simulink model "QPSKMODEM"  (R2020b)
settings: Solver=VariableStepAuto  StartTime=0.0  StopTime=inf  RelTol=1e-3
model workspace (MAT data in the model file):
  BitRate = 20480
  CoreFreq = 40960
  RCF_Rolloff_factor = 0.1
  SampleRateQPSK = 819200
undefined symbols (not defined in the file): fdesignblkfcn, gcbh, random
libraries: simulink_extras x9, simulink x6, commfilt2 x4, dspsrcs4 x3, commrfcorlib x2, commutil2 x2, dspmathops x2, commrandsrc3 x1, commsink2 x1, commchan3 x1
(part 1 of 2)
settings Model: OrderedModelArguments=off  Creator=Unknown Username  LastModifiedBy=AlexKurash
settings DataIOCC: ReturnWorkspaceOutputs=off
settings DebuggingCC: ParameterOverflowMsg=none  ArithmeticOperatorsInVariantConditions=warning
settings SFSimCC: SimUseLocalCustomCode=off  CustomCodeUndefinedFunction=UseInterfaceOnly
settings RTWCC: RTWUseLocalCustomCode=off

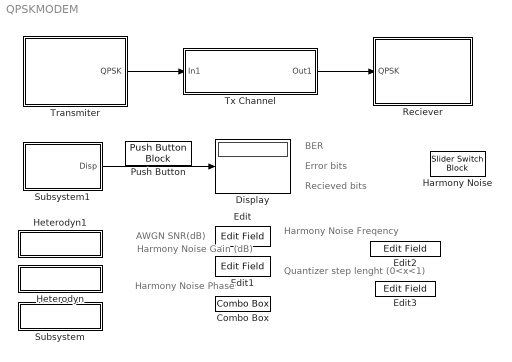
== system QPSKMODEM ==
  note: BER
  note: Error bits
  note: Recieved bits
  note: AWGN SNR(dB)
  note: Harmony Noise
      | Gain (dB)
  note: Harmony Noise
      | Phase
  note: Harmony Noise
      | Freqency
  note: Quantizer step lenght (0<x<1)
  Combo Box : ComboBox  LabelPosition=Hide  SelectedLabel=45deg
      settings: Values={{'0deg', '10deg', '20deg', '30deg', '45deg', '90deg', '180deg'}, [0 0.174533 0.349066 0.523598 0.785398 1.570796 3.141592]}
  Display : Display
  Edit{,1..3} (4 alike) : EditField  LabelPosition=Hide  ShowInitialText=on  Alignment=Center
  Harmony Noise : SliderSwitchBlock
      settings: Values={{'Off', 'On'}, [0 1]}
  Heterodyn : Subsystem
      mask Display:
      | color('red');
      | disp('Heterodyn')
  Heterodyn1 : Subsystem
      mask Display:
      | color('red');
      | disp('Syncronization')
  Push Button : PushButtonBlock  ButtonText=RESET
  Reciever : Subsystem
      mask Display:
      | color('purple');
      | disp('OQPSK \n RECIEVER')
      | color('black');
  Subsystem : Subsystem
      mask Display:
      | color('red');
      | disp('Dbit Generator')
  Subsystem1 : Subsystem
      mask Display:
      | color('red')
      | 
      | disp('Graphics\n and \n BER calculation')
  Transmiter : Subsystem
      mask Display:
      | color('blue');
      | disp('OQPSK \n TRANSMITER')
      | color('black');
  Tx Channel : Subsystem
      mask Display:
      | plot(-10,-10,110, 110,[05 15 10 10 05 10 18 14 13 7.5 13 41 44 47 50 53 57 ...
      | 59 100-[13 7.5 13 14 18 10 5 10 10 15 5]],[70 70 70 85 92 85 79 82 90 88.5 ...
      | 90 90 87 93 87 93 87 90 90 88.5 90 82 79 85 92 85 70 70 70]);
      | disp('CHANNEL');
  wires:
  Subsystem1/1(Disp) -> Display/1
  Transmiter/1(QPSK) -> Tx Channel/1(In1)
  Tx Channel/1(Out1) -> Reciever/1(QPSK)

== system QPSKMODEM/Heterodyn ==
  Local Oscillator : dspsrcs4/Sine Wave  Amplitude=0.707  Frequency=CoreFreq  Phase=pi/2  SampleMode=Discrete  OutComplex=Real  CompMethod=Trigonometric fcn  TableSize=Speed  SampleTime=1/SampleRateQPSK  SamplesPerFrame=1  ResetState=Restart at time zero  OutputFrames=off  dataType=double  wordLen=16  udDataType=sfix(16)  fracBitsMode=Best precision  numFracBits=15  OutDataTypeStr=double  LastOutDataTypeStr=double
  Local Oscillator1 : dspsrcs4/Sine Wave  Amplitude=0.707  Frequency=CoreFreq  Phase=0  SampleMode=Discrete  OutComplex=Real  CompMethod=Trigonometric fcn  TableSize=Speed  SampleTime=1/SampleRateQPSK  SamplesPerFrame=1  ResetState=Restart at time zero  OutputFrames=off  dataType=double  wordLen=16  udDataType=sfix(16)  fracBitsMode=Best precision  numFracBits=15  OutDataTypeStr=double  LastOutDataTypeStr=double
  tag scope: Heterodyn_COS=global, Heterodyn_SIN=global
  wires:
  Local Oscillator/1 -> [Heterodyn_COS]
  Local Oscillator1/1 -> [Heterodyn_SIN]

== system QPSKMODEM/Heterodyn1 ==
  Clock : simulink_extras/Flip Flops/Clock  period=2/BitRate
  tag scope: CLK=global
  wires:
  Clock/1 -> [CLK]

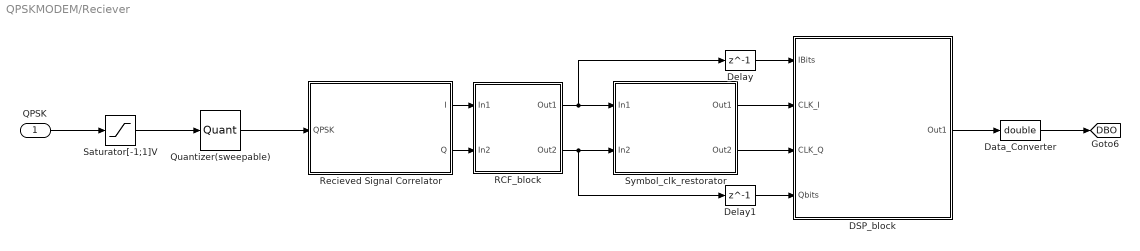
== system QPSKMODEM/Reciever ==
  QPSK : Inport
  DSP_block : Subsystem
      mask Display:
      | color('red');
      | disp('Digital \n Signal \n Processing')
      | color('black');
      | port_label('input',3,'CLK_Q')
      | port_label('input',2,'CLK_I')
      | port_label('input',1,'I_bits')
      | port_label('input',4,'Q_bits')
      | port_label('output',1,'DBit_code')
  Data_Converter : DataTypeConversion  OutDataTypeStr=double
  Delay : Delay  DelayLength=1  InitialCondition=0  SampleTime=1/BitRate
  Delay1 : Delay  DelayLength=1  InitialCondition=0  SampleTime=1/BitRate
  Quantizer(sweepable) : Quantizer  QuantizationInterval=1/8  LinearizeAsGain=off
  RCF_block : Subsystem
      mask Display:
      | color('red');
      | disp('Filtration')
      | color('black');
      | port_label('input',1,'I')
      | port_label('input',2,'Q')
      | port_label('output',1,'I')
      | port_label('output',2,'Q')
  "Recieved Signal Correlator " : Subsystem
      mask Display:
      | color('red');
      | disp('Correlation')
      | color('black');
      | port_label('input',1,'OPSK')
      | port_label('output',1,'I')
      | port_label('output',2,'Q')
  Saturator[-1;1]V : Saturate  UpperLimit=1  LowerLimit=-1
  Symbol_clk_restorator : Subsystem
      mask Display:
      | color('red');
      | disp('Syncronization \n restoration')
      | color('black');
      | port_label('input',1,'s(t_I)')
      | port_label('output',1,'CLK_I')
      | 
      | port_label('input',2,'s(t_Q)')
      | port_label('output',2,'CLK_Q')
  tag scope: DBO=global
  wires:
  Data_Converter/1 -> [DBO]
  "Recieved Signal Correlator "/1(I) -> RCF_block/1(In1)
  "Recieved Signal Correlator "/2(Q) -> RCF_block/2(In2)
  RCF_block/1(Out1) -> Delay/1, Symbol_clk_restorator/1(In1)
  RCF_block/2(Out2) -> Delay1/1, Symbol_clk_restorator/2(In2)
  Symbol_clk_restorator/1(Out1) -> DSP_block/2(CLK_I)
  Symbol_clk_restorator/2(Out2) -> DSP_block/3(CLK_Q)
  Delay/1 -> DSP_block/1(IBits)
  Delay1/1 -> DSP_block/4(Qbits)
  Saturator[-1;1]V/1 -> Quantizer(sweepable)/1
  DSP_block/1(Out1) -> Data_Converter/1
  Quantizer(sweepable)/1 -> "Recieved Signal Correlator "/1(QPSK)
  QPSK/1 -> Saturator[-1;1]V/1

== system QPSKMODEM/Subsystem ==
  Bernoulli Binary Generator : commrandsrc3/Bernoulli Binary Generator  ProbabilityOfZero=0.5  SeedSource=Auto  Seed=random  SampleTime=1/BitRate  SamplesPerFrame=1  OutputDataType=double  SimulateUsing=Interpreted execution
  tag scope: DB=global
  wires:
  Bernoulli Binary Generator/1 -> [DB]

== system QPSKMODEM/Subsystem1 ==
  Reciever : Subsystem
      mask Display: disp('Transmitter \n Diagrams')
  Subsystem : Subsystem
      mask Display: disp('BER \n Calculation')
  Transmiter : Subsystem
      mask Display: disp('Reciever \n Diagrams')
  spectre : Subsystem
      mask Display: disp('Signals\nSpectrum')
  spectre1 : Subsystem
      mask Display: disp('Constellation \n Diagramm')
  Disp : Outport  VectorParamsAs1DForOutWhenUnconnected=off
  wires:
  Subsystem/1(Out1) -> Disp/1

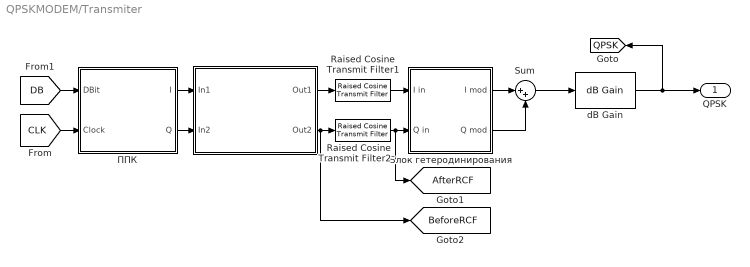
== system QPSKMODEM/Transmiter ==
  " " : Subsystem
      mask Display:
      | color('red');
      | disp('Signal Level \n Coder')
      | color('black');
      | port_label('input',1,'Odd_in')
      | port_label('input',2,'Even_in')
      | port_label('output',1,'Odd_out')
      | port_label('output',2,'Even_out')
  Raised Cosine Transmit Filter1 : commfilt2/Raised Cosine Transmit Filter  filtType=Square root  R=RCF_Rolloff_factor  filtSpan=10  N=(SampleRateQPSK/BitRate)/4  filterGain=3  RateOptions=Allow multirate processing  framing=Mute  checkCoeff=off  variableName=rcTxFilt1  checkGain=Normalized  sampMode=Mute  saveAsFlag=0  currentFiltSpan=10  D=(10)/2  launchFVT=on  roundingMode=Floor  overflowMode=off  coeffDataTypeStr=Inherit: Same word length as input  coeffMin=[]  coeffMax=[]  coeffLastDataTypeStr=Inherit: Same word length as input  outputDataTypeStr=Inherit: Same as accumulator  outputMin=[]  outputMax=[]  outputLastDataTypeStr=Inherit: Same as accumulator
  Raised Cosine Transmit Filter2 : commfilt2/Raised Cosine Transmit Filter  filtType=Square root  R=RCF_Rolloff_factor  filtSpan=10  N=(SampleRateQPSK/BitRate)/4  filterGain=3  RateOptions=Allow multirate processing  framing=Mute  checkCoeff=off  variableName=rcTxFilt2  checkGain=Normalized  sampMode=Mute  saveAsFlag=0  currentFiltSpan=10  D=(10)/2  launchFVT=on  roundingMode=Floor  overflowMode=off  coeffDataTypeStr=Inherit: Same word length as input  coeffMin=[]  coeffMax=[]  coeffLastDataTypeStr=Inherit: Same word length as input  outputDataTypeStr=Inherit: Same as accumulator  outputMin=[]  outputMax=[]  outputLastDataTypeStr=Inherit: Same as accumulator
  Sum : Sum  Inputs=|++
  dB Gain : dspmathops/dB Gain  dB=5  intype=Power
      settings: SourceProductBaseCode=DS
  "Блок гетеродинирования " : Subsystem
      mask Display:
      | color('red');
      | disp('Hyterodination')
      | color('black');
      | port_label('input',1,'Odd')
      | port_label('input',2,'Even')
      | port_label('output',1,'I')
      | port_label('output',2,'Q')
  ППК : Subsystem
      mask Display:
      | color('red');
      | disp('Serial-to-Parallel')
      | color('black');
      | port_label('input',1,'Dbit')
      | port_label('input',2,'CLK')
      | port_label('output',1,'Odd')
      | port_label('output',2,'Even')
  QPSK : Outport  VectorParamsAs1DForOutWhenUnconnected=off
  tag scope: AfterRCF=global, BeforeRCF=global, QPSK=global
  wires:
  [DB] -> ППК/1(DBit)
  [CLK] -> ППК/2(Clock)
  ППК/1(I) -> " "/1(In1)
  ППК/2(Q) -> " "/2(In2)
  "Блок гетеродинирования "/1(I mod) -> Sum/1
  "Блок гетеродинирования "/2(Q mod) -> Sum/2
  " "/1(Out1) -> Raised Cosine Transmit Filter1/1
  " "/2(Out2) -> [BeforeRCF], Raised Cosine Transmit Filter2/1
  Raised Cosine Transmit Filter1/1 -> "Блок гетеродинирования "/1(I in)
  Raised Cosine Transmit Filter2/1 -> [AfterRCF], "Блок гетеродинирования "/2(Q in)
  dB Gain/1 -> QPSK/1, [QPSK]
  Sum/1 -> dB Gain/1

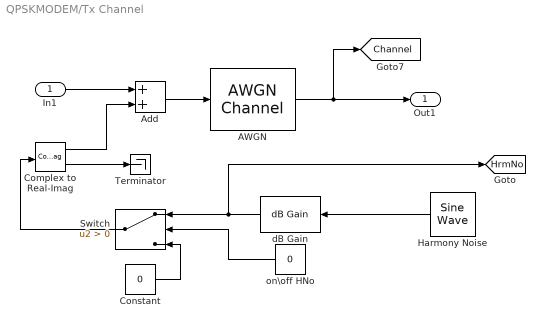
== system QPSKMODEM/Tx Channel ==
  In1 : Inport
  AWGN : commchan3/AWGN Channel  InputProcessing=Columns as channels (frame based)  seed=1  noiseMode="Signal to noise ratio  (SNR)"  EbNodB=20  EsNodB=10  SNRdB=20  bitsPerSym=2  Ps=200  Tsym=0.5/BitRate  variance=1
  Add : Sum
  Complex to Real-Imag : ComplexToRealImag
  Constant : Constant  Value=0
  Harmony Noise : dspsrcs4/Sine Wave  Amplitude=0.707  Frequency=41000  Phase=0.785398  SampleMode=Discrete  OutComplex=Real  CompMethod=Trigonometric fcn  TableSize=Speed  SampleTime=1/SampleRateQPSK  SamplesPerFrame=1  ResetState=Restart at time zero  OutputFrames=off  dataType=double  wordLen=16  udDataType=sfix(16)  fracBitsMode=Best precision  numFracBits=15  OutDataTypeStr=double  LastOutDataTypeStr=double
  Switch : Switch  Criteria=u2 > Threshold
  Terminator : Terminator
  dB Gain : dspmathops/dB Gain  dB=0  intype=Power
      settings: SourceProductBaseCode=DS
  on\off HNo : Constant  Value=0
  Out1 : Outport
  tag scope: Channel=global, HrmNo=global
  wires:
  dB Gain/1 -> [HrmNo], Switch/1
  on\off HNo/1 -> Switch/2
  In1/1 -> Add/1
  Add/1 -> AWGN/1
  Switch/1 -> Complex to Real-Imag/1
  AWGN/1 -> [Channel], Out1/1
  Complex to Real-Imag/1 -> Add/2
  Harmony Noise/1 -> dB Gain/1
  Complex to Real-Imag/2 -> Terminator/1
  Constant/1 -> Switch/3

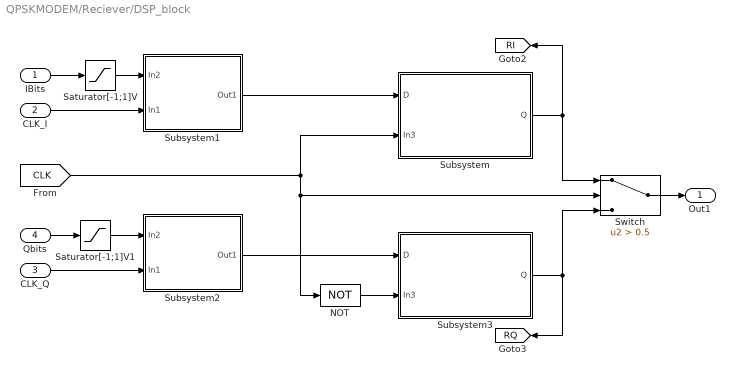
== system QPSKMODEM/Reciever/DSP_block ==
  IBits : Inport
  CLK_I : Inport  Port=2
  CLK_Q : Inport  Port=3
  Qbits : Inport  Port=4
  NOT : Logic  Operator=NOT  AllPortsSameDT=off  OutDataTypeStr=boolean
  Saturator[-1;1]V : Saturate  UpperLimit=1  LowerLimit=-1
  Saturator[-1;1]V1 : Saturate  UpperLimit=1  LowerLimit=-1
  Subsystem : Subsystem
      mask Display:
      | color('red');
      | disp('Bits \n Restoration \n device')
      | color('black');
      | port_label('output',1,'Bits')
      | port_label('input',1,'s(t)')
      | port_label('input',2,'CLK')
  Subsystem1 : Subsystem
      mask Display:
      | color('red');
      | disp('Treshold \n decision \n device')
      | color('black');
      | port_label('output',1,'Bits')
      | port_label('input',1,'s(t)')
      | port_label('input',2,'CLK')
  Subsystem2 : Subsystem
      mask Display:
      | color('red');
      | disp('Treshold \n decision \n device')
      | color('black');
      | port_label('output',1,'Bits')
      | port_label('input',1,'s(t)')
      | port_label('input',2,'CLK')
  Subsystem3 : Subsystem
      mask Display:
      | color('red');
      | disp('Bits \n Restoration \n device')
      | color('black');
      | port_label('output',1,'Bits')
      | port_label('input',1,'s(t)')
      | port_label('input',2,'CLK')
  Switch : Switch  Criteria=u2 > Threshold  Threshold=0.5
  Out1 : Outport
  tag scope: RI=global, RQ=global
  wires:
  Subsystem1/1(Out1) -> Subsystem/1(D)
  Subsystem2/1(Out1) -> Subsystem3/1(D)
  CLK_I/1 -> Subsystem1/2(In1)
  Subsystem3/1(Q) -> Switch/3, [RQ]
  Switch/1 -> Out1/1
  IBits/1 -> Saturator[-1;1]V/1
  Qbits/1 -> Saturator[-1;1]V1/1
  NOT/1 -> Subsystem3/2(In3)
  CLK_Q/1 -> Subsystem2/2(In1)
  [CLK] -> Switch/2, NOT/1, Subsystem/2(In3)
  Subsystem/1(Q) -> Switch/1, [RI]
  Saturator[-1;1]V/1 -> Subsystem1/1(In2)
  Saturator[-1;1]V1/1 -> Subsystem2/1(In2)

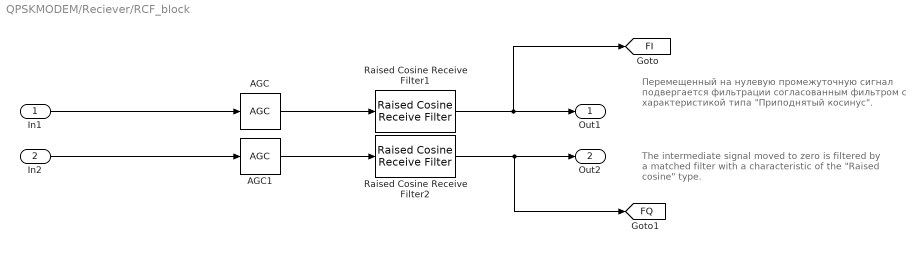
== system QPSKMODEM/Reciever/RCF_block ==
  note: The intermediate signal moved to zero is
      | filtered by a matched filter with a characteristic
      | of the "Raised cosine" type.
  note: Перемещенный на нулевую промежуточную
      | сигнал подвергается фильтрации согласованным
      | фильтром с характеристикой типа "Приподнятый косинус".
  In1 : Inport
  In2 : Inport  Port=2
  AGC : commrfcorlib/AGC  LegacyMode=off  DetectorMethod=Rectifier  LoopMethod=Linear  UpdatePeriod=100  StepSize=0.1  AdaptationStepSize=0.01  DesiredOutputPower=0.1  AveragingLength=100  MaximumGain=30  MaxPowerGain=0  GainOutputPort=off  InputPowerOutputPort=off  SimulateUsing=Interpreted execution
  AGC1 : commrfcorlib/AGC  LegacyMode=off  DetectorMethod=Rectifier  LoopMethod=Linear  UpdatePeriod=100  StepSize=0.1  AdaptationStepSize=0.01  DesiredOutputPower=0.1  AveragingLength=100  MaximumGain=30  MaxPowerGain=0  GainOutputPort=off  InputPowerOutputPort=off  SimulateUsing=Interpreted execution
  Raised Cosine Receive Filter1 : commfilt2/Raised Cosine Receive Filter  filtType=Square root  R=RCF_Rolloff_factor  filtSpan=10  N=(SampleRateQPSK/BitRate)  downFactor=(SampleRateQPSK/BitRate)/8  downOffset=0  filterGain=1  RateOptions=Allow multirate processing  framing=Mute  checkCoeff=off  variableName=rcRxFilt1  currentFiltSpan=10  D=(10)/2  inputOffset=0  sampMode=Mute  saveAsFlag=0  rateMode=Downsampling  checkGain=Normalized  launchFVT=on  roundingMode=Floor  overflowMode=off  coeffDataTypeStr=Inherit: Same word length as input  coeffMin=[]  coeffMax=[]  coeffLastDataTypeStr=Inherit: Same word length as input  accumDataTypeStr=Inherit: Same as product output  accumLastDataTypeStr=Inherit: Same as product output  outputDataTypeStr=Inherit: Same as accumulator  outputMin=[]  outputMax=[]  outputLastDataTypeStr=Inherit: Same as accumulator
  Raised Cosine Receive Filter2 : commfilt2/Raised Cosine Receive Filter  filtType=Square root  R=RCF_Rolloff_factor  filtSpan=10  N=(SampleRateQPSK/BitRate)  downFactor=(SampleRateQPSK/BitRate)/8  downOffset=0  filterGain=1  RateOptions=Allow multirate processing  framing=Mute  checkCoeff=off  variableName=rcRxFilt2  currentFiltSpan=10  D=(10)/2  inputOffset=0  sampMode=Mute  saveAsFlag=0  rateMode=Downsampling  checkGain=Normalized  launchFVT=on  roundingMode=Floor  overflowMode=off  coeffDataTypeStr=Inherit: Same word length as input  coeffMin=[]  coeffMax=[]  coeffLastDataTypeStr=Inherit: Same word length as input  accumDataTypeStr=Inherit: Same as product output  accumLastDataTypeStr=Inherit: Same as product output  outputDataTypeStr=Inherit: Same as accumulator  outputMin=[]  outputMax=[]  outputLastDataTypeStr=Inherit: Same as accumulator
  Out1 : Outport  VectorParamsAs1DForOutWhenUnconnected=off
  Out2 : Outport  Port=2  VectorParamsAs1DForOutWhenUnconnected=off
  tag scope: FI=global, FQ=global
  wires:
  In2/1 -> AGC1/1
  In1/1 -> AGC/1
  Raised Cosine Receive Filter1/1 -> [FI], Out1/1
  Raised Cosine Receive Filter2/1 -> [FQ], Out2/1
  AGC/1 -> Raised Cosine Receive Filter1/1
  AGC1/1 -> Raised Cosine Receive Filter2/1

== system QPSKMODEM/Reciever/Recieved Signal Correlator  ==
  note: Mixing the signals in this block causes
      | the signal spectrum to move to the
      | zero intermediate frequency
  note: В результате смешения сигналов
      | в этом блоке происходит перемещение
      | спектральной составляющей сигнала
      | на нулевую промежуточную частоту.
  QPSK : Inport
  Product : Product  Inputs=**
  Product1 : Product  Inputs=**
  I : Outport  VectorParamsAs1DForOutWhenUnconnected=off
  Q : Outport  Port=2  VectorParamsAs1DForOutWhenUnconnected=off
  tag scope: HI=global, HQ=global, Rec=global
  wires:
  Product/1 -> [HI], I/1
  Product1/1 -> Q/1, [HQ]
  QPSK/1 -> Product1/2, Product/1, [Rec]
  [Heterodyn_SIN] -> Product1/1
  [Heterodyn_COS] -> Product/2

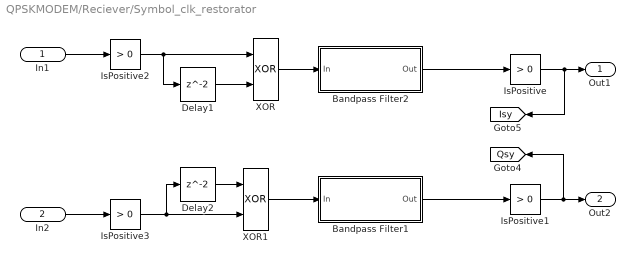
== system QPSKMODEM/Reciever/Symbol_clk_restorator ==
  In1 : Inport
  In2 : Inport  Port=2
  Bandpass Filter1 : Subsystem  DialogController=fdesignblkfcn  InitFcn=fdesignblkfcn(gcbh, {'InitFcn'});  mask(Bandpass Filter){}
      mask help: Design a bandpass filter
      settings: CopyFcn=fdesignblkfcn(gcbh, {'CopyFcn'});
      mask Help: helpview(mapfilelocation('dsp'), 'dspbandpassfilter');
      mask Display: disp('Bandpass');
  Bandpass Filter2 : Subsystem  DialogController=fdesignblkfcn  InitFcn=fdesignblkfcn(gcbh, {'InitFcn'});  mask(Bandpass Filter){}
      mask help: Design a bandpass filter
      settings: CopyFcn=fdesignblkfcn(gcbh, {'CopyFcn'});
      mask Help: helpview(mapfilelocation('dsp'), 'dspbandpassfilter');
      mask Display: disp('Bandpass');
  Delay1 : Delay  InitialCondition=0
  Delay2 : Delay  InitialCondition=0
  IsPositive{,1..3} (4 alike) : simulink/Logic and Bit Operations/Compare To Zero  relop=>  OutDataTypeStr=boolean
  XOR : Logic  Operator=XOR  IconShape=distinctive  AllPortsSameDT=off  OutDataTypeStr=fixdt(1,16)
  XOR1 : Logic  Operator=XOR  IconShape=distinctive  AllPortsSameDT=off  OutDataTypeStr=fixdt(1,16)
  Out1 : Outport  VectorParamsAs1DForOutWhenUnconnected=off
  Out2 : Outport  Port=2  VectorParamsAs1DForOutWhenUnconnected=off
  tag scope: Isy=global, Qsy=global
  wires:
  Bandpass Filter2/1(Out) -> IsPositive/1
  Delay1/1 -> XOR/2
  Bandpass Filter1/1(Out) -> IsPositive1/1
  IsPositive/1 -> Out1/1, [Isy]
  IsPositive1/1 -> Out2/1, [Qsy]
  Delay2/1 -> XOR1/1
  In2/1 -> IsPositive3/1
  IsPositive2/1 -> XOR/1, Delay1/1
  IsPositive3/1 -> Delay2/1, XOR1/2
  In1/1 -> IsPositive2/1
  XOR/1 -> Bandpass Filter2/1(In)
  XOR1/1 -> Bandpass Filter1/1(In)

== system QPSKMODEM/Subsystem1/Reciever ==
  "Dbit code , I and Q signals" : Scope  NumInputPorts=3
  OQPSK signal with I and Q channels : Scope  NumInputPorts=3
  wires:
  [IS] -> OQPSK signal with I and Q channels/1
  [QB] -> "Dbit code , I and Q signals"/2
  [IB] -> "Dbit code , I and Q signals"/3
  [DB] -> "Dbit code , I and Q signals"/1
  [QS] -> OQPSK signal with I and Q channels/2
  [QPSK] -> OQPSK signal with I and Q channels/3

== system QPSKMODEM/Subsystem1/Subsystem ==
  Delay1 : Delay  DelayLength=1  InitialCondition=0  SampleTime=1/BitRate
  Delay2 : Delay  DelayLength=16  InitialCondition=0  SampleTime=1/BitRate
  Error Rate Calculation : commsink2/Error Rate Calculation  N=0  st_delay=15  cp_mode=Entire frame  subframe=[]  PMode=Port  WsName=ErrorVec  RsMode2=on  stop=on  numErr=1e6  maxBits=1e6
  One : Constant  Value=0
  Scope : Scope  NumInputPorts=2
  Out1 : Outport  VectorParamsAs1DForOutWhenUnconnected=off
  wires:
  [DBO] -> Delay1/1
  [DB] -> Delay2/1
  Error Rate Calculation/1 -> Out1/1
  Delay2/1 -> Scope/1, Error Rate Calculation/1
  One/1 -> Error Rate Calculation/3
  Delay1/1 -> Scope/2, Error Rate Calculation/2

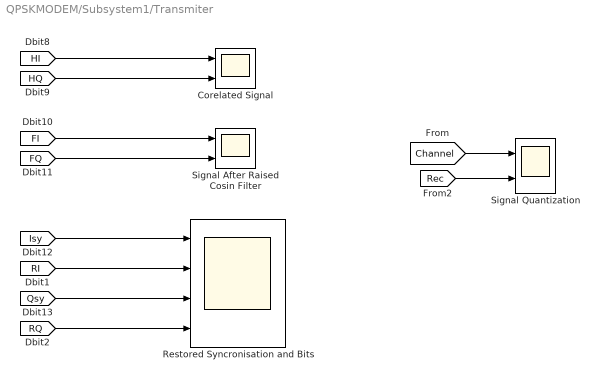
== system QPSKMODEM/Subsystem1/Transmiter ==
  Corelated Signal : Scope  NumInputPorts=2
  Restored Syncronisation and Bits : Scope  NumInputPorts=4
  Signal After Raised Cosin Filter : Scope  NumInputPorts=2
  Signal Quantization : Scope  NumInputPorts=2
  wires:
  [RI] -> Restored Syncronisation and Bits/2
  [Isy] -> Restored Syncronisation and Bits/1
  [Qsy] -> Restored Syncronisation and Bits/3
  [RQ] -> Restored Syncronisation and Bits/4
  [HI] -> Corelated Signal/1
  [HQ] -> Corelated Signal/2
  [FI] -> Signal After Raised Cosin Filter/1
  [FQ] -> Signal After Raised Cosin Filter/2
  [Rec] -> Signal Quantization/2
  [Channel] -> Signal Quantization/1

== system QPSKMODEM/Subsystem1/spectre ==
  Matrix Concatenate : Concatenate  Mode=Multidimensional array  ConcatenateDimension=2
  Spectrum of bits after RCF : SpectrumAnalyzer
  Tx and Rx spectrum : SpectrumAnalyzer  NumInputPorts=3
  wires:
  [QPSK] -> Tx and Rx spectrum/1  "Transmited Signal"
  [HrmNo] -> Tx and Rx spectrum/2  "Harmony Noise Spectrum"
  [Channel] -> Tx and Rx spectrum/3  "Recieved Signal"
  [AfterRCF] -> Matrix Concatenate/1  "Signal after RCF"
  [BeforeRCF] -> Matrix Concatenate/2  "Signal before RCF"
  Matrix Concatenate/1 -> Spectrum of bits after RCF/1

== system QPSKMODEM/Subsystem1/spectre1 ==
  Constellation Diagram : ConstellationDiagram
  Real-Imag to Complex : RealImagToComplex
  wires:
  [FI] -> Real-Imag to Complex/1
  Real-Imag to Complex/1 -> Constellation Diagram/1
  [FQ] -> Real-Imag to Complex/2

== system QPSKMODEM/Transmiter/  ==
  In1 : Inport
  In2 : Inport  Port=2
  U-B converter : commutil2/Unipolar to Bipolar Converter  M=2  polarity=Positive  dataType=double
  U-B converter1 : commutil2/Unipolar to Bipolar Converter  M=2  polarity=Positive  dataType=Inherit via internal rule
  Out1 : Outport  VectorParamsAs1DForOutWhenUnconnected=off
  Out2 : Outport  Port=2  VectorParamsAs1DForOutWhenUnconnected=off
  wires:
  U-B converter1/1 -> Out2/1
  U-B converter/1 -> Out1/1
  In1/1 -> U-B converter/1
  In2/1 -> U-B converter1/1

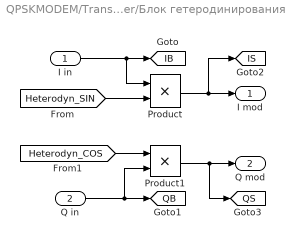
== system QPSKMODEM/Transmiter/Блок гетеродинирования  ==
  I in : Inport
  Q in : Inport  Port=2
  Product : Product  Inputs=**
  Product1 : Product
  I mod : Outport  VectorParamsAs1DForOutWhenUnconnected=off
  Q mod : Outport  Port=2  VectorParamsAs1DForOutWhenUnconnected=off
  tag scope: IB=global, IS=global, QB=global, QS=global
  wires:
  [Heterodyn_COS] -> Product1/1
  [Heterodyn_SIN] -> Product/2
  I in/1 -> [IB], Product/1
  Q in/1 -> [QB], Product1/2
  Product/1 -> I mod/1, [IS]
  Product1/1 -> [QS], Q mod/1

== system QPSKMODEM/Transmiter/ППК ==
  DBit : Inport
  Clock : Inport  Port=2
  Cast To Double : DataTypeConversion  OutMin=-1  OutMax=+1  OutDataTypeStr=double
  Cast To Double1 : DataTypeConversion  OutMin=-1  OutMax=+1  OutDataTypeStr=double
  Блок растяжения импульсов : Subsystem
      mask Display:
      | color('red');
      | disp('Symbol stretching')
      | color('black');
      | port_label('input',1,'Odd_in')
      | port_label('input',2,'Even_in')
      | port_label('input',3,'CLK')
      | port_label('output',1,'Odd_out')
      | port_label('output',2,'Even_out')
  Демультиплексор : Subsystem
      mask Display:
      | color('red');
      | disp('Demux')
      | color('black');
      | port_label('input',1,'D')
      | port_label('input',2,'CLK')
      | port_label('output',1,'Odd_out')
      | port_label('output',2,'Even_out')
  I : Outport  VectorParamsAs1DForOutWhenUnconnected=off
  Q : Outport  Port=2  VectorParamsAs1DForOutWhenUnconnected=off
  wires:
  Cast To Double/1 -> I/1
  Cast To Double1/1 -> Q/1
  Clock/1 -> Блок растяжения импульсов/3(Clock), Демультиплексор/2(Code)
  DBit/1 -> Демультиплексор/1(D)
  Демультиплексор/1(A1) -> Блок растяжения импульсов/1(First bit)
  Демультиплексор/2(A2) -> Блок растяжения импульсов/2(Second Bit)
  Блок растяжения импульсов/2(Q) -> Cast To Double1/1
  Блок растяжения импульсов/1(I) -> Cast To Double/1

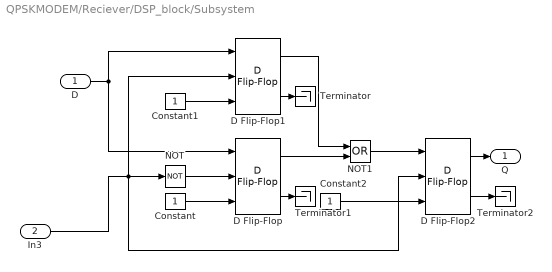
== system QPSKMODEM/Reciever/DSP_block/Subsystem ==
  D : Inport
  In3 : Inport  Port=2
  Constant : Constant
  Constant1 : Constant
  Constant2 : Constant
  D Flip-Flop : simulink_extras/Flip Flops/D Flip-Flop
  D Flip-Flop1 : simulink_extras/Flip Flops/D Flip-Flop
  D Flip-Flop2 : simulink_extras/Flip Flops/D Flip-Flop
  NOT : Logic  Operator=NOT  AllPortsSameDT=off  OutDataTypeStr=boolean
  NOT1 : Logic  Operator=OR  AllPortsSameDT=off  OutDataTypeStr=boolean
  Terminator : Terminator
  Terminator1 : Terminator
  Terminator2 : Terminator
  Q : Outport
  wires:
  D Flip-Flop1/1 -> NOT1/1
  Constant2/1 -> D Flip-Flop2/3
  D Flip-Flop2/1 -> Q/1
  Constant/1 -> D Flip-Flop/3
  Constant1/1 -> D Flip-Flop1/3
  D Flip-Flop/1 -> NOT1/2
  NOT/1 -> D Flip-Flop/2
  NOT1/1 -> D Flip-Flop2/1
  D/1 -> D Flip-Flop/1, D Flip-Flop1/1
  In3/1 -> D Flip-Flop1/2, D Flip-Flop2/2, NOT/1
  D Flip-Flop1/2 -> Terminator/1
  D Flip-Flop/2 -> Terminator1/1
  D Flip-Flop2/2 -> Terminator2/1

== system QPSKMODEM/Reciever/DSP_block/Subsystem1 ==
  In2 : Inport
  In1 : Inport  Port=2
  IsPositive : simulink/Logic and Bit Operations/Compare To Zero  relop=>  OutDataTypeStr=boolean
  Product : Product
  Out1 : Outport  VectorParamsAs1DForOutWhenUnconnected=off
  wires:
  In1/1 -> Product/2
  In2/1 -> Product/1
  IsPositive/1 -> Out1/1
  Product/1 -> IsPositive/1

== system QPSKMODEM/Reciever/DSP_block/Subsystem2 ==
  In2 : Inport
  In1 : Inport  Port=2
  IsPositive : simulink/Logic and Bit Operations/Compare To Zero  relop=>  OutDataTypeStr=boolean
  Product : Product
  Out1 : Outport  VectorParamsAs1DForOutWhenUnconnected=off
  wires:
  In1/1 -> Product/2
  In2/1 -> Product/1
  IsPositive/1 -> Out1/1
  Product/1 -> IsPositive/1

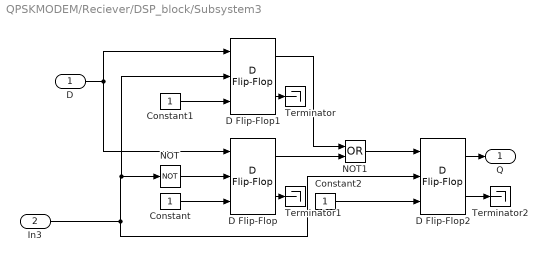
== system QPSKMODEM/Reciever/DSP_block/Subsystem3 ==
  D : Inport
  In3 : Inport  Port=2
  Constant : Constant
  Constant1 : Constant
  Constant2 : Constant
  D Flip-Flop : simulink_extras/Flip Flops/D Flip-Flop
  D Flip-Flop1 : simulink_extras/Flip Flops/D Flip-Flop
  D Flip-Flop2 : simulink_extras/Flip Flops/D Flip-Flop
  NOT : Logic  Operator=NOT  AllPortsSameDT=off  OutDataTypeStr=boolean
  NOT1 : Logic  Operator=OR  AllPortsSameDT=off  OutDataTypeStr=boolean
  Terminator : Terminator
  Terminator1 : Terminator
  Terminator2 : Terminator
  Q : Outport
  wires:
  D Flip-Flop1/1 -> NOT1/1
  Constant2/1 -> D Flip-Flop2/3
  D Flip-Flop2/1 -> Q/1
  Constant/1 -> D Flip-Flop/3
  In3/1 -> D Flip-Flop2/2, D Flip-Flop1/2, NOT/1
  Constant1/1 -> D Flip-Flop1/3
  D Flip-Flop/1 -> NOT1/2
  NOT/1 -> D Flip-Flop/2
  NOT1/1 -> D Flip-Flop2/1
  D/1 -> D Flip-Flop/1, D Flip-Flop1/1
  D Flip-Flop1/2 -> Terminator/1
  D Flip-Flop/2 -> Terminator1/1
  D Flip-Flop2/2 -> Terminator2/1

== system QPSKMODEM/Reciever/Symbol_clk_restorator/Bandpass Filter1 ==
  In : Inport
  Generated Filter Block : DiscreteFir  Tag=BlockMethodSubSystem  Coefficients=[1.33291293613741489e-06 -3.71729674503269073e-06 -2.55982433042465191e-06 -2.3244966415084971e-06 -2.0722245476230491e-06 -1.50854830451986809e-06 -5.72891685133694265e-07 6.65656947025783295e-07 2.04911167673330056e-06 3.35197704869231731e-06 4.32055999851877012e-06 4.71151414744170765e-06 4.34530519577557304e-06 3.14564616485739826e-06 1.17753788969815406e-06 -1.34636792999603235e-06 -4.07375681599398936e-06 -6.56025667124246123e-06 -8.32830846950749775e-06 -8.95475221998336354e-06 -8.14768533239771636e-06 -5.8259593796378098e-06 -2.15690289505963077e-06 2.42768022547142276e-06 7.27866172757355486e-06 1.16014189686021614e-05 1.4586450061584313e-05 1.55339848578051398e-05 1.40086871319831641e-05 9.92697107453206786e-06 3.64974736138616162e-06 -4.0649354262165857e-06 -1.20930363766651291e-05 -1.91304462997007023e-05 -2.38835268125860489e-05 -2.52595024430426598e-05 -2.26226286098086369e-05 -1.59322907835080267e-05 -5.8230715145782389e-06 6.42819751348861043e-06 1.90338354835750395e-05 2.99458667561533163e-05 3.71668264264164933e-05 3.90947632637926118e-05 3.48304656309026539e-05 2.44069925721513521e-05 8.88074976814050208e-06 -9.73414589850726173e-06 -2.8703505146679707e-05 -4.49514345798067013e-05 -5.55378556077206398e-05 -5.81583294413739419e-05 -5.15899573692238451e-05 -3.59995863972453691e-05 -1.30518143912198537e-05 1.42212426546720768e-05 4.17898549903912732e-05 6.5194728062666646e-05 8.02417564023146776e-05 8.37132768455236273e-05 7.39872746307630041e-05 5.14473521720787956e-05 1.85967920979521701e-05 -2.01545172868308598e-05 -5.90584458982579085e-05 -9.18331833531083172e-05 -0.000112657573781342699 -0.000117152435651038335 -0.000103214617718458597 -7.15506955373990968e-05 -2.57990541768897453e-05 2.78269231657254816e-05 8.13363112470276986e-05 0.0001261150273754031 0.000154270437507517491 0.000159970002534428777 0.00014054476822755396 9.71680622123971961e-05 3.49586967850069982e-05 -3.7543941000230478e-05 -0.000109502657605406337 -0.00016935774900787799 -0.000206639206936389138 -0.000213732395340630627 -0.000187313692288571508 -0.000129193034557493038 -4.6391288403871765e-05 4.96216147612247059e-05 0.000144455257338812571 0.000222909604845972491 0.000271354986875024426 0.000280031031321154467 0.000244867170379394253 0.000168524530020135638 6.0410638870396045e-05 -6.43757209733221333e-05 -0.000187090084176245834 -0.000288104887231354051 -0.000349987496540658588 -0.000360426665037735664 -0.000314524064490422387 -0.000216037916425287387 -7.73228293229287196e-05 8.21099480516207248e-05 0.000238265479255448081 0.000366218525796791925 0.000444025874211647319 0.000456397849892745469 0.000397523992669530988 0.000272553928949029168 9.74142095137955536e-05 -0.000103101460023173242 -0.000298765733713606246 -0.000458409264960771593 -0.000554817290313541853 -0.000569267289588973389 -0.000494969698399205056 -0.000338796460210581977 -0.000120935877677477211 0.000127591262896608324 0.00036926412578416754 0.000565661311626165808 0.000683492929052940327 0.000700137004399498759 0.000607768671461196282 0.000415354283618889816 0.000148089637033452096 -0.000155766743255090394 -0.000450282512722346225 -0.000688725149942851053 -0.000830901168858613607 -0.000849816758113741688 -0.000736574061871812509 -0.000502642351229692116 -0.000179016349192079923 0.000187749991531884695 0.000542151484787903228 0.000828060744966827196 0.000997539170306453379 0.00101875684840367522 0.000881728783528820843 0.000600863951675842172 0.000213781511948922374 -0.000223583327422953622 -0.000644974405495246737 -0.000983780922026523128 -0.00118348871639559401 -0.001206986428611575 -0.00104321153086955323 -0.000709975363607827934 -0.000252363502226554475 0.00026321835999364477 0.000758594950399557252 0.00115560522993273245 0.00138836042753224349 0.00141405651139719316 0.00122059160224736009 0.000829656527376232324 0.000294642223916765896 -0.000306507808665003583 -0.000882570147217811782 -0.00134282083196826229 -0.00161125044688458646 -0.0016389999409642073 ...(+10366 chars)]
  Out : Outport  VectorParamsAs1DForOutWhenUnconnected=off
  wires:
  In/1 -> Generated Filter Block/1
  Generated Filter Block/1 -> Out/1
